simulink model "jooooo"  (R2022a)
settings: Solver=VariableStepAuto  StartTime=0.0  StopTime=4  RelTol=1e-3
libraries: simulink x1
settings Model: Creator=gbour  LastModifiedBy=gbour

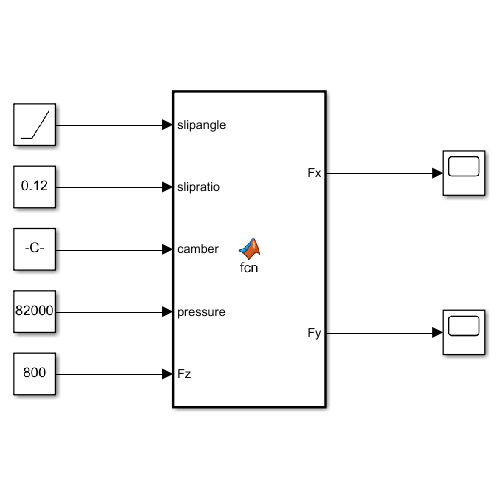
[thumbnail: Simulink's stored preview of the top-level diagram]
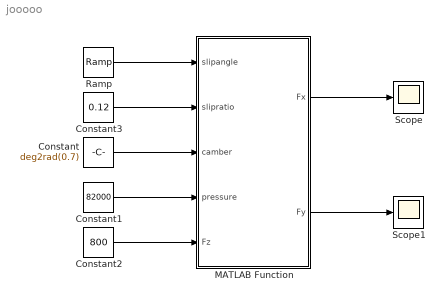
== system jooooo ==
  Constant : Constant  Value=deg2rad(0.7)
  Constant1 : Constant  Value=82000
  Constant2 : Constant  Value=800
  Constant3 : Constant  Value=0.12
  MATLAB Function : MATLAB Function  TreatAsAtomicUnit=on
  Ramp : simulink/Sources/Ramp  slope=0.1  start=0  InitialOutput=-0.2
  Scope : Scope
  Scope1 : Scope
  wires:
  MATLAB Function/1(Fx) -> Scope/1
  MATLAB Function/2(Fy) -> Scope1/1
  Constant/1 -> MATLAB Function/3(camber)
  Constant1/1 -> MATLAB Function/4(pressure)
  Constant2/1 -> MATLAB Function/5(Fz)
  Ramp/1 -> MATLAB Function/1(slipangle)
  Constant3/1 -> MATLAB Function/2(slipratio)

== matlab function jooooo/MATLAB Function ==
  data: slipangle input; Fx output; slipratio input; camber input; pressure input; Fz input; Fy output
function [Fx, Fy] = fcn(slipangle, slipratio, camber, pressure, Fz)

coder.extrinsic('magicformula.v62.eval')

tireSide = 0;
Fx = 0;
Fy = 0;

[Fx, Fy, ~, ~] = magicformula.v62.eval(slipangle, slipratio, camber, pressure, Fz, tireSide);

end
